simulink model "task3"  (R2018a)
settings: Solver=ode3  StartTime=0.0  StopTime=8.5  FixedStep=0.01  RelTol=1e-3
settings Model: Creator=richardkong  LastModifiedBy=richardkong

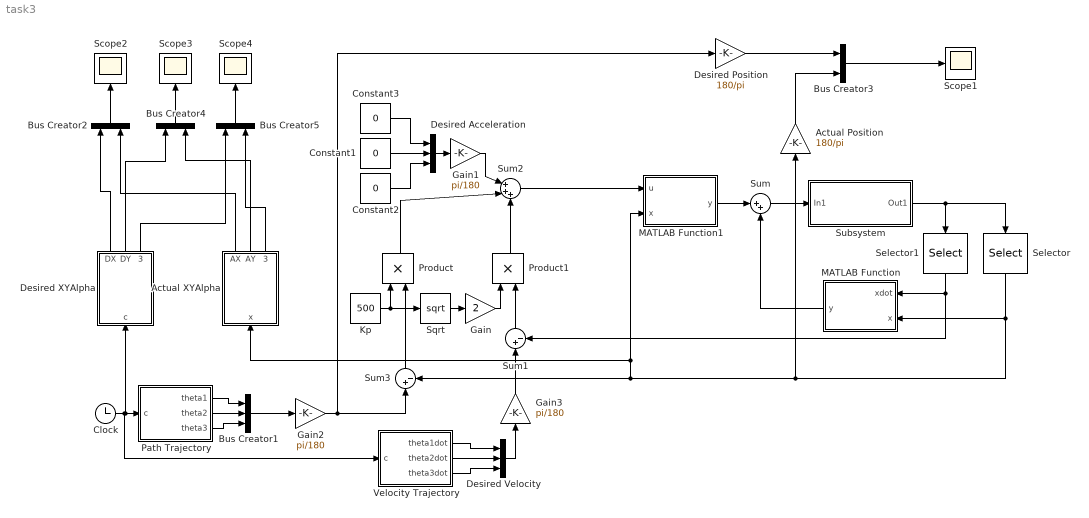
== system task3 ==
  Actual XYAlpha : MATLAB Function  TreatAsAtomicUnit=on
  Actual Position : Gain  Gain=180/pi
  Bus Creator1 : BusCreator  Inputs=3
  Bus Creator{2..5} (4 alike) : BusCreator  Inputs=2
  Clock : Clock
  Constant1 : Constant  Value=0
  Constant2 : Constant  Value=0
  Constant3 : Constant  Value=0
  Desired Acceleration : BusCreator  Inputs=3
  Desired Velocity : BusCreator  Inputs=3
  Desired XYAlpha : MATLAB Function  TreatAsAtomicUnit=on
  Desired Position : Gain  Gain=180/pi
  Gain : Gain  Gain=2
  Gain1 : Gain  Gain=pi/180
  Gain2 : Gain  Gain=pi/180
  Gain3 : Gain  Gain=pi/180
  Kp : Constant  Value=500
  MATLAB Function : MATLAB Function  TreatAsAtomicUnit=on
  MATLAB Function1 : MATLAB Function  TreatAsAtomicUnit=on
  Path Trajectory : MATLAB Function  TreatAsAtomicUnit=on
  Product : Product
  Product1 : Product
  Scope{1..4} (4 alike) : Scope
  Selector : Selector  InputPortWidth=6  IndexOptions=Index vector (dialog)  Indices=[1 3 5]  OutputSizes=1
  Selector1 : Selector  InputPortWidth=6  IndexOptions=Index vector (dialog)  Indices=[2 4 6]  OutputSizes=1
  Sqrt : Sqrt  SaturateOnIntegerOverflow=on
  Subsystem : Subsystem
  Sum : Sum  Inputs=|++
  Sum1 : Sum  Inputs=|+-
  Sum2 : Sum  Inputs=|+++
  Sum3 : Sum  Inputs=|+-
  Velocity Trajectory : MATLAB Function  TreatAsAtomicUnit=on
  wires:
  Selector1/1 -> Sum1/2, MATLAB Function/1(xdot)
  Sum1/1 -> Product1/2
  Product/1 -> Sum2/2
  Constant1/1 -> Desired Acceleration/2
  Selector/1 -> Actual Position/1, Sum3/2, Actual XYAlpha/1(x), MATLAB Function1/2(x), MATLAB Function/2(x)
  MATLAB Function1/1(y) -> Sum/1
  Sum/1 -> Subsystem/1(In1)
  Sum2/1 -> MATLAB Function1/1(u)
  Constant2/1 -> Desired Acceleration/3
  Kp/1 -> Sqrt/1, Product/1
  MATLAB Function/1(y) -> Sum/2
  Sum3/1 -> Product/2
  Sqrt/1 -> Gain/1
  Subsystem/1(Out1) -> Selector/1, Selector1/1
  Desired Velocity/1 -> Gain3/1
  Gain/1 -> Product1/1
  Product1/1 -> Sum2/3
  Desired Acceleration/1 -> Gain1/1
  Gain1/1 -> Sum2/1
  Gain2/1 -> Desired Position/1, Sum3/1
  Gain3/1 -> Sum1/1
  Constant3/1 -> Desired Acceleration/1
  Bus Creator1/1 -> Gain2/1
  Path Trajectory/3(theta3) -> Bus Creator1/3
  Path Trajectory/1(theta1) -> Bus Creator1/1
  Path Trajectory/2(theta2) -> Bus Creator1/2
  Bus Creator3/1 -> Scope1/1
  Clock/1 -> Desired XYAlpha/1(c), Path Trajectory/1(c), Velocity Trajectory/1(c)
  Desired Position/1 -> Bus Creator3/1
  Actual Position/1 -> Bus Creator3/2
  Bus Creator2/1 -> Scope2/1
  Desired XYAlpha/1(DX) -> Bus Creator2/1
  Actual XYAlpha/1(AX) -> Bus Creator2/2
  Bus Creator4/1 -> Scope3/1
  Desired XYAlpha/2(DY) -> Bus Creator4/1
  Actual XYAlpha/2(AY) -> Bus Creator4/2
  Bus Creator5/1 -> Scope4/1
  Desired XYAlpha/3(Dalpha) -> Bus Creator5/1
  Actual XYAlpha/3(Aalpha) -> Bus Creator5/2
  Velocity Trajectory/2(theta2dot) -> Desired Velocity/2
  Velocity Trajectory/3(theta3dot) -> Desired Velocity/3
  Velocity Trajectory/1(theta1dot) -> Desired Velocity/1

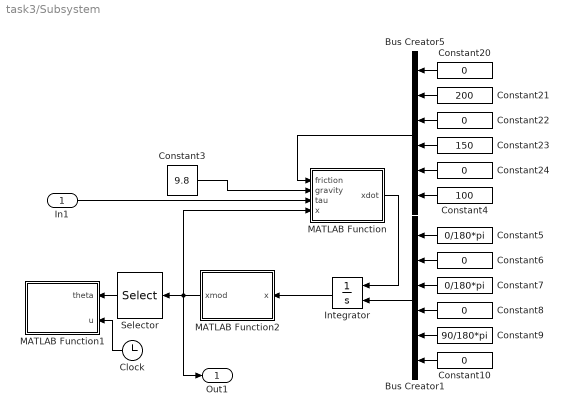
== system task3/Subsystem ==
  In1 : Inport
  Bus Creator1 : BusCreator  Inputs=6
  Bus Creator5 : BusCreator  Inputs=6
  Clock : Clock
  Constant{6,8,10,20,22,24} (6 alike) : Constant  Value=0
  Constant21 : Constant  Value=200
  Constant23 : Constant  Value=150
  Constant3 : Constant  Value=9.8
  Constant4 : Constant  Value=100
  Constant5 : Constant  Value=0/180*pi
  Constant7 : Constant  Value=0/180*pi
  Constant9 : Constant  Value=90/180*pi
  Integrator : Integrator  InitialConditionSource=external  InitialCondition=[1/18*pi;0;1/9*pi;0;1/6*pi;0]
  MATLAB Function : MATLAB Function  TreatAsAtomicUnit=on
  MATLAB Function1 : MATLAB Function  TreatAsAtomicUnit=on
  MATLAB Function2 : MATLAB Function  TreatAsAtomicUnit=on
  Selector : Selector  InputPortWidth=6  IndexOptions=Index vector (dialog)  Indices=[1 3 5]  OutputSizes=1
  Out1 : Outport
  wires:
  Constant10/1 -> Bus Creator1/6
  Constant22/1 -> Bus Creator5/3
  Constant21/1 -> Bus Creator5/2
  Constant24/1 -> Bus Creator5/5
  Constant23/1 -> Bus Creator5/4
  Constant9/1 -> Bus Creator1/5
  Integrator/1 -> MATLAB Function2/1(x)
  Constant7/1 -> Bus Creator1/3
  Bus Creator5/1 -> MATLAB Function/1(friction)
  Constant5/1 -> Bus Creator1/1
  MATLAB Function/1(xdot) -> Integrator/1
  Constant6/1 -> Bus Creator1/2
  Bus Creator1/1 -> Integrator/2
  Constant4/1 -> Bus Creator5/6
  Constant3/1 -> MATLAB Function/2(gravity)
  Selector/1 -> MATLAB Function1/1(theta)
  Constant20/1 -> Bus Creator5/1
  Constant8/1 -> Bus Creator1/4
  In1/1 -> MATLAB Function/3(tau)
  MATLAB Function2/1(xmod) -> MATLAB Function/4(x), Out1/1, Selector/1
  Clock/1 -> MATLAB Function1/2(u)

== matlab function task3/Subsystem/MATLAB Function1 ==
  data: theta input; u input
function animate(theta,u)
%#codegen
coder.extrinsic('saveas');
coder.extrinsic('num2str');
u = int16( u / 0.01) + 1;
theta1 = theta(1);
theta2 = theta(2);
theta3 = theta(3);
%hold off
T_0 = eye(4);
hold off
l1 = 4;
l2 = 3;
l3 = 2;
point1=[[0,0,0];[4,0,0]];
point2 = [[0,0,0];[3,0,0]];
point3 = [[0,0,0];[2,0,0]];

T_01 = [cos(theta1) -sin(theta1) 0 0; sin(theta1) cos(theta1) 0 0; 0 0 1 0; 0 0 0 1];
T_12 = [cos(theta2) -sin(theta2) 0 l1; sin(theta2) cos(theta2) 0 0; 0 0 1 0; 0 0 0 1];
T_23 = [cos(theta3) -sin(theta3) 0 l2; sin(theta3) cos(theta3) 0 0; 0 0 1 0; 0 0 0 1];

point1 = [point1 [1;1]];
point2 = [point2 [1;1]];
point3 = [point3 [1;1]];
     
point1 = (T_0 * T_01 * point1')';
       
point2 = (T_0 * T_01 * T_12 * point2')';

point3 = (T_0 * T_01 * T_12 * T_23 * point3')';

plot(point1(:,1),point1(:,2));
hold on
plot(point2(:,1),point2(:,2));
grid on
plot(point3(:,1),point3(:,2));
grid on
axis([-15 15 -15 15 -15 15]);
xlabel('X');
ylabel('Y');
title('Kp = 500, Kv = 44.72');
if rem(u, 5) == 1
    %saveas(gcf,['/Users/richardkong/Desktop/Robotics/Final/Trajectory/',num2str(u,'%04d')],'png');
end
end

== matlab function task3/Subsystem/MATLAB Function ==
  data: friction input; gravity input; tau input; xdot output; x input
function xdot = fcn(friction, gravity, tau, x)
%#codegen
theta1 = x(1);
theta_1 = x(2);
theta2 = x(3);
theta_2 = x(4);
theta3 = x(5);
theta_3 = x(6);

f_1 = friction(2);
f_2 = friction(4);
f_3 = friction(6);

g = gravity;
tau1 = tau(1);
tau2 = tau(2);
tau3 = tau(3);

m1 = 20;
m2 = 15;
m3 = 10;
l1 = 4;
l2 = 3;
l3 = 2;
Izz1 = 0.5;
Izz2 = 0.2;
Izz3 = 0.1;

M11 = m3 * (l1^2 + l2^2 + l3^2/4 + 2*l1*l2*cos(theta2) + l2*l3*cos(theta3) + l1*l3*cos(theta2 + theta3)) + m2 * (l1^2 + l2^2/4 + l1*l2*cos(theta2)) + m1 * l1^2/4 + Izz1 + Izz2 + Izz3;
M12 = m3 * (l2^2 + l3^2/4 + l1*l2*cos(theta2) + l2*l3*cos(theta3) + l1*l3/2*cos(theta2 + theta3)) + m2 * (l2^2/4 + l1*l2/2*cos(theta2)) + Izz2 + Izz3;
M13 = m3 * (l3^2/4 + l2*l3/2*cos(theta3) + l1*l3/2*cos(theta2 + theta3)) + Izz3;
M21 = M12;
M22 = m3 * (l2^2 + l3^2/4 + l2*l3*cos(theta3)) + m2 * l2^2/4 + Izz2 + Izz3;
M23 = m3 * (l3^2/4 + l2*l3/2*cos(theta3)) + Izz3;
M31 = M13;
M32 = M23;
M33 = m3 * l3^2/4 + Izz3;

C12 = m3 * (-l1*l2*sin(theta2) - l1*l3/2*sin(theta2 + theta3)) + m2 * (-l1*l2/2*sin(theta2));
C21 = -C12;
C13 = m3 * (-l2*l3/2*sin(theta3) - l1*l3/2*sin(theta2 + theta3));
C31 = -C13;
C23 = m3 * (-l2 * l3 / 2 * sin(theta3));
C32 = -C23;

B11 = 2 * (m3 * (-l1*l2*sin(theta2)-l1*l3/2*sin(theta2 + theta3)) + m2 * (-l1 * l2/2 * sin(theta2)));
B12 = 2 * (m3 * (-l2*l3/2*sin(theta3)-l1*l3/2*sin(theta2 + theta3)));
B13 = B12;
B22 = -2 * (m3 * l2 * l3 / 2 * sin(theta3));
B23 = B22;
B31 = -1 * B23;

G1 = cos(theta1)*l1/2*m1*g + (cos(theta1+theta2)*l2/2+cos(theta1)*l1)*m2*g + (cos(theta1 + theta2 + theta3)*l3/2 + cos(theta1 + theta2)*l2 + cos(theta1)*l1) * m3*g;
G2 = cos(theta1+theta2)*l2/2*m2*g + (cos(theta1 + theta2 + theta3)*l3/2 + cos(theta1 + theta2)*l2) * m3*g;
G3 = cos(theta1 + theta2 + theta3)*l3/2 * m3 * g;

M = [M11 M12 M13; M21 M22 M23; M31 M32 M33];
C = [0 C12 C13; C21 0 C23; C31 C32 0];
B = [B11 B12 B13; 0 B22 B23; B31 0 0];
G = [G1; G2; G3];

ans = [tau1-f_1*theta_1;tau2-f_2*theta_2;tau3-f_3*theta_3] - C * [theta_1^2;theta_2^2;theta_3^2] - B * [theta_1 * theta_2;theta_1 * theta_3;theta_2 * theta_3] - G;
E = inv(M) * ans;
theta_11 = E(1);
theta_22 = E(2);
theta_33 = E(3);

xdot = [theta_1; theta_11; theta_2; theta_22; theta_3; theta_33];
end

== matlab function task3/Subsystem/MATLAB Function2 ==
  data: x input; xmod output
function xmod = fcn(x)
q1 = x(1);
q2 = x(3);
q3 = x(5);
%q1 = atan2(sin(q1), cos(q1));
q2 = atan2(sin(q2), cos(q2));
q3 = atan2(sin(q3), cos(q3));
xmod = [q1;x(2);q2;x(4);q3;x(6)];

== matlab function task3/MATLAB Function ==
  data: xdot input; x input; y output
function y = CBG(xdot, x)

m1 = 20;
m2 = 15;
m3 = 10;
l1 = 4;
l2 = 3;
l3 = 2;
g = 9.8;

theta1 = x(1);
theta2 = x(2);
theta3 = x(3);

theta_1 = xdot(1);
theta_2 = xdot(2);
theta_3 = xdot(3);

C12 = m3 * (-l1*l2*sin(theta2) - l1*l3/2*sin(theta2 + theta3)) + m2 * (-l1*l2/2*sin(theta2));
C21 = -C12;
C13 = m3 * (-l2*l3/2*sin(theta3) - l1*l3/2*sin(theta2 + theta3));
C31 = -C13;
C23 = m3 * (-l2 * l3 / 2 * sin(theta3));
C32 = -C23;

B11 = 2 * (m3 * (-l1*l2*sin(theta2)-l1*l3/2*sin(theta2 + theta3)) + m2 * (-l1 * l2/2 * sin(theta2)));
B12 = 2 * (m3 * (-l2*l3/2*sin(theta3)-l1*l3/2*sin(theta2 + theta3)));
B13 = B12;
B22 = -2 * (m3 * l2 * l3 / 2 * sin(theta3));
B23 = B22;
B31 = -1 * B23;

G1 = cos(theta1)*l1/2*m1*g + (cos(theta1+theta2)*l2/2+cos(theta1)*l1)*m2*g + (cos(theta1 + theta2 + theta3)*l3/2 + cos(theta1 + theta2)*l2 + cos(theta1)*l1) * m3*g;
G2 = cos(theta1+theta2)*l2/2*m2*g + (cos(theta1 + theta2 + theta3)*l3/2 + cos(theta1 + theta2)*l2) * m3*g;
G3 = cos(theta1 + theta2 + theta3)*l3/2 * m3 * g;

C = [0 C12 C13; C21 0 C23; C31 C32 0];
B = [B11 B12 B13; 0 B22 B23; B31 0 0];
G = [G1; G2; G3];

y = C * [theta_1^2;theta_2^2;theta_3^2] + B * [theta_1 * theta_2;theta_1 * theta_3;theta_2 * theta_3] + G;

== matlab function task3/MATLAB Function1 ==
  data: u input; y output; x input
function y = Mass(u, x)

theta1 = x(1);
theta2 = x(2);
theta3 = x(3);

m1 = 20;
m2 = 15;
m3 = 10;
l1 = 4;
l2 = 3;
l3 = 2;
Izz1 = 0.5;
Izz2 = 0.2;
Izz3 = 0.1;

M11 = m3 * (l1^2 + l2^2 + l3^2/4 + 2*l1*l2*cos(theta2) + l2*l3*cos(theta3) + l1*l3*cos(theta2 + theta3)) + m2 * (l1^2 + l2^2/4 + l1*l2*cos(theta2)) + m1 * l1^2/4 + Izz1 + Izz2 + Izz3;
M12 = m3 * (l2^2 + l3^2/4 + l1*l2*cos(theta2) + l2*l3*cos(theta3) + l1*l3/2*cos(theta2 + theta3)) + m2 * (l2^2/4 + l1*l2/2*cos(theta2)) + Izz2 + Izz3;
M13 = m3 * (l3^2/4 + l2*l3/2*cos(theta3) + l1*l3/2*cos(theta2 + theta3)) + Izz3;
M21 = M12;
M22 = m3 * (l2^2 + l3^2/4 + l2*l3*cos(theta3)) + m2 * l2^2/4 + Izz2 + Izz3;
M23 = m3 * (l3^2/4 + l2*l3/2*cos(theta3)) + Izz3;
M31 = M13;
M32 = M23;
M33 = m3 * l3^2/4 + Izz3;

M = [M11 M12 M13; M21 M22 M23; M31 M32 M33];
y = M * u;

== matlab function task3/Path Trajectory ==
  data: c input; theta1 output; theta2 output; theta3 output
function [theta1, theta2, theta3] = fcn(c)
x = load('trajectory.mat');
x = x.s;
q1 = x(1,:);
q2 = x(2,:);
q3 = x(3,:);
i = c/0.01 + 1;
index = int16(i);
if (index > int16(801))
    index = int16(801);
end
theta1 = q1(index);
theta2 = q2(index);
theta3 = q3(index);

== matlab function task3/Velocity Trajectory ==
  data: c input; theta1dot output; theta2dot output; theta3dot output
function [theta1dot, theta2dot, theta3dot] = fcn(c)
x = load('velocity.mat');
x = x.b;
q1 = x(1,:);
q2 = x(2,:);
q3 = x(3,:);
i = c/0.01 + 1;
index = int16(i);
if (index > int16(801))
    index = int16(1);
end
theta1dot = q1(index);
theta2dot = q2(index);
theta3dot = q3(index);

== matlab function task3/Desired XYAlpha ==
  data: c input; DX output; DY output; Dalpha output
function [DX, DY, Dalpha] = fcn(c)
x = load('xyalpha.mat');
x = x.y;
X_ = x(1,:);
Y_ = x(2,:);
alpha_ = x(3,:);
i = c/0.01 + 1;
index = int16(i);
if (index > int16(801))
    index = int16(801);
end
DX = X_(index);
DY = Y_(index);
Dalpha = alpha_(index);

== matlab function task3/Actual XYAlpha ==
  data: x input; AX output; AY output; Aalpha output
function [AX, AY, Aalpha] = fcn(x)
theta1 = x(1);
theta2 = x(2);
theta3 = x(3);
l1 = 4;
l2 = 3;
l3 = 2;
AX = l3 * cos(theta1 + theta2 + theta3) + l2 * cos(theta2 + theta1) + l1 * cos(theta1);
AY = l3 * sin(theta1 + theta2 + theta3) + l2 * sin(theta2 + theta1) + l1 * sin(theta1);
Aalpha = atan2(AY, AX);
